simulink model "part2"  (R2025a)
settings: Solver=ode4  StartTime=0.0  StopTime=500  FixedStep=0.1  RelTol=1e-3
values from neighbouring files (symbols this model uses):
  A_f = diag([1/t1 1/t2 1/t3])    [reference_model.m]
  A_w = [zeros(3,3), eye(3); -omega_ekf^2, -2*lambda_ekf*omega_ekf]    [kalman.m]
  Aw = [zeros(3,3), eye(3); -omega*omega, -2*lambda*omega]    [observer.m]
  B_ekf = [zeros(6,3);zeros(3,3); zeros(3,3);M_inv]    [kalman.m]
  Cw = [zeros(3,3), eye(3)]    [observer.m]
  D_diag = D    [observer.m]
  E_ekf = [E_w zeros(6,3) ... (first row only)    [kalman.m]
  G = zeros(3,3)    [kalman.m]
  Gamma = diag([w1^2, w2^2, w3^2])    [reference_model.m]
  H_ekf = [C_w eye(3) zeros(3,3) zeros(3,3)]    [kalman.m]
  h_ekf = 0.1    [kalman.m]
  K1 = [diag([k1, k2, k3]); diag([k4, k5, k6])]    [observer.m]
  K2 = diag([k7, k8, k9])    [observer.m]
  K3 = 0.1* K4    [observer.m]
  K4 = diag([M_diag(1,1), M_diag(1,1), M_diag(1,1)])*1e-1    [observer.m]
  K_w_ekf = diag(Kwi)    [kalman.m]
  Kd = diag([Kd_t(1,1), Kd_t(2,2), Kd_t(3,3)])    [PID.m]
  Ki = diag([Ki_t(1,1), Ki_t(2,2), Ki_t(3,3)])    [PID.m]
  Kp = diag([Kp_t(1,1), Kp_t(2,2), Kp_t(3,3)])    [PID.m]
  lambda_ekf = diag(zeta)    [kalman.m]
  M_diag = [Mtot(1,1), 0, 0 ... (first row only)    [observer.m]
  M_inv = inv(M_3)    [kalman.m]    (also in observer.m = inv(M_diag))
  mu = 0.001    [init.m]
  mu_direction = 0.03    [init.m]
  Omega = diag([2*zeta1*w1, 2*zeta2*w2, 2*zeta3*w3])    [reference_model.m]
  omega_ekf = diag([w, w, w])    [kalman.m]
  P_0 = eye(15)    [kalman.m]
  Q_ekf = diag([0.001, 0.001, 0.001, 1e8, 1e8, 1e9])    [kalman.m]
  R_ekf = diag([1, 5, 0.01])    [kalman.m]
  rate = [rate(1), rate(2), rate(2), rate(3), rate(4),rate(4), rate(5), rate(5)]    [thrust_allocation.m]
  rotationspeed = [0 rotationspeed(1) 0 rotationspeed(2) rotationspeed(3)]    [thrust_allocation.m]
  step1 = 50    [reference_model.m]
  step2 = 1.4    [reference_model.m]
  step3 = 1.2    [reference_model.m]
  T_b_ekf = 1000*diag([1, 1, 1])    [kalman.m]
  Tb_inv = inv(Tb)    [observer.m]
  thrust = [thrust(1), thrust(2), thrust(2), thrust(3), thrust(4), thrust(4), thrust(5), thrust(5)]    [thrust_allocation.m]
  U_10 = 10    [init.m]
  U_angle = 180    [init.m]
  U_mean = U_10*(5/2)*sqrt(K)*log(z/z0)    [init.m]
  W = diag([10, 1, 1, 10, 1, 1, 1, 1])    [thrust_allocation.m]
  w = 0.005    [init.m]    (also in kalman.m = 0.698131700798)
  x_0 = zeros(1,15)    [kalman.m]
  xpos = [thrusters.xposition]    [thrust_allocation.m]
  ypos = [thrusters.yposition]    [thrust_allocation.m]
undefined symbols (not defined in the file or in its folder): alpha, C_pitch, C_roll, C_yaw, Cx, Cy, Cz, Hoerner, thrusters, vessel, wind_coeff
libraries: marine_gnc x9, simulink x8, dspsigops x3, marine_hydro x2, simulink_extras x2
(part 1 of 2)
settings Model: Creator=jonbjor  LastModifiedBy=audun
settings DataIOCC: ReturnWorkspaceOutputs=off
settings DebuggingCC: AlgebraicLoopMsg=none  UnconnectedInputMsg=warning  UnconnectedOutputMsg=warning  UnconnectedLineMsg=warning  ArithmeticOperatorsInVariantConditions=warning
settings ModelReferenceCC: EnableRefExpFcnMdlSchedulingChecks=on
settings SFSimCC: SimUseLocalCustomCode=off  CustomCodeUndefinedFunction=UseInterfaceOnly
settings RTWCC: RTWUseLocalCustomCode=off  GPUComputeCapability=3.5  DLArmComputeVersion=19.05

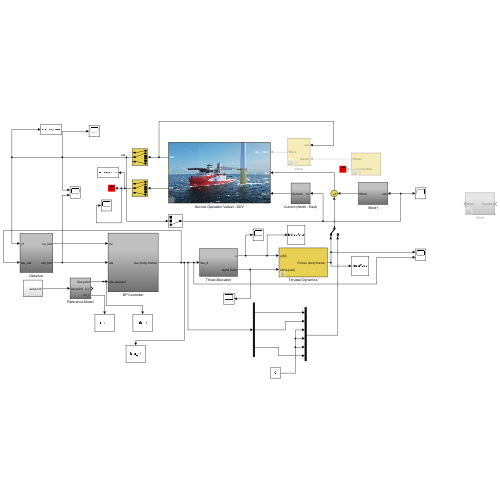
[thumbnail: Simulink's stored preview of the top-level diagram]
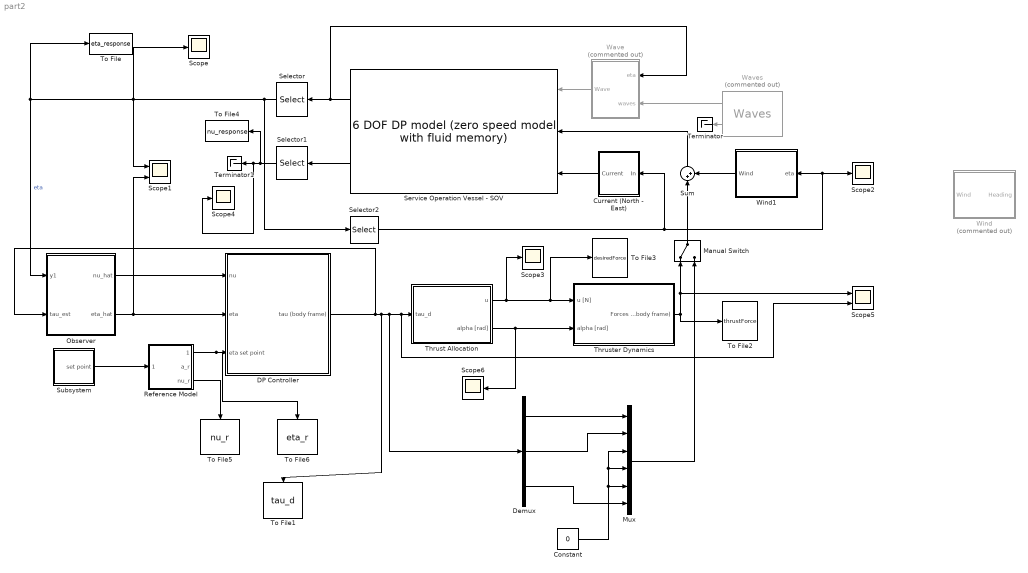
== system part2 ==
  Constant : Constant  Value=0
  Current (North - East) : Subsystem
  DP Controller : Subsystem
  Demux : Demux  Outputs=3
  Manual Switch : ManualSwitch
  Mux : Mux  Inputs=6
  Observer : Subsystem
  Reference Model : Subsystem
  Scope{,2..4,6} (5 alike) : Scope
      Scope settings: ActiveDisplayYMinimum=-447.3734  ActiveDisplayYMaximum=52.18517  DataLoggingVariableName=ScopeData6
      Scope2 settings: ActiveDisplayYMinimum=-0.38407  ActiveDisplayYMaximum=3.45663  DataLoggingVariableName=ScopeData2
      Scope3 settings: ActiveDisplayYMinimum=-11170.42553  ActiveDisplayYMaximum=24574.49173
      Scope4 settings: ActiveDisplayYMinimum=-1.13887  ActiveDisplayYMaximum=0.80341  DataLoggingVariableName=ScopeData2
      Scope6 settings: ActiveDisplayYMinimum=-0.17279  ActiveDisplayYMaximum=1.76453
  Scope1 : Scope  NumInputPorts=2
      settings: ActiveDisplayYMinimum=-560.03158  ActiveDisplayYMaximum=66.18767
  Scope5 : Scope  NumInputPorts=2
      settings: ActiveDisplayYMinimum=-36332.60871  ActiveDisplayYMaximum=326993.47836  DataLoggingVariableName=ScopeData3
  Selector : Selector  InputPortWidth=6  IndexOptions=Index vector (dialog)  Indices=[1 2 6]  OutputSizes=1
  Selector1 : Selector  InputPortWidth=6  IndexOptions=Index vector (dialog)  Indices=[1 2 6]  OutputSizes=1
  Selector2 : Selector  InputPortWidth=3  IndexOptions=Index vector (dialog)  Indices=[3]  OutputSizes=1
  Service Operation Vessel - SOV : marine_hydro/Hydro Library/6 DOF DP model  (zero speed model with fluid memory)  ABC=vesselABC  rho=1025  Axc=0.9*vessel.main.T*vessel.main.B  Ayc=0.9*vessel.main.T*vessel.main.Lpp  CX=1  CY_2D=Hoerner(vessel.main.B,vessel.main.T)  Bv=vessel.Bv  mask(6 DOF zero speed model){}
      link override "Integrator1 ": InitialCondition=nu0
      link override Integrator2: InitialCondition=eta0
      settings: SourceProductName=MSS Hydro
      mask Display:
      | image('SOV.jpg');
      | color('white'); port_label('output', 1, 'eta')
      | color('white'); port_label('output', 2, 'nu')
      | color('white'); port_label('input', 1, 'tau_wave')
      | color('white'); port_label('input', 2, 'tau')
      | color('white'); port_label('input', 3, 'nu_c')
  Subsystem : Subsystem
  Sum : Sum  Inputs=|++
  Terminator : Terminator
  Terminator1 : Terminator
  Thrust Allocation : Subsystem
  Thruster Dynamics : Subsystem  mask{thrusterfault=off}
      mask prompts: thrusterfault "Fault on thruster #2 and #4?"
  To File : ToFile  Filename=eta_response  MatrixName=eta_response
  To File1 : ToFile  Filename=tau_d  MatrixName=tau_d
  To File2 : ToFile  Filename=thrustForce  MatrixName=thrustForce
  To File3 : ToFile  Filename=desiredForce  MatrixName=desiredForce
  To File4 : ToFile  Filename=nu_response  MatrixName=nu_response
  To File5 : ToFile  Filename=nu_r  MatrixName=nu_r
  To File6 : ToFile  Filename=eta_r  MatrixName=eta_r
  Wave : Subsystem  Commented=on  mask{waveforces=on}
      mask prompts: waveforces "Waveforces enabled"
  Waves : marine_gnc/Environment/Waves/Waves  Commented=on  spectrum_type=ITTC  disp_flag=on  plot_spectrum=off  plot_realization=off  hs=2.5  omega_peak=2*pi/9  psi_mean=0  gamma=-1  spread=2  depth=inf  nfreq=20  ndir=10  energylim=0.005  freq_cutoff=3  dir_cutoff=0  rand_seed=123  rand_freq=on  rand_dir=on  Zeta_a=0  Omega=0  Phase=0  Wavenum=0  Psi=0
      link override Psi: Value=-6*pi/8*ones(1,38)
      settings: SourceProductName=MSS GNC
  Wind : Subsystem  Commented=on
  Wind1 : Subsystem
  wires:
  Service Operation Vessel - SOV/2 -> Selector1/1
  Service Operation Vessel - SOV/1 -> Wave/1(eta), Selector/1
  Current (North - East)/1(Current) -> Service Operation Vessel - SOV/3
  Wave/1(Wave) -> Service Operation Vessel - SOV/1
  Waves/1 -> Wave/2(waves)
  Waves/2 -> Terminator/1
  Sum/1 -> Service Operation Vessel - SOV/2
  Selector/1 -> Selector2/1, Scope/1, To File/1, Observer/1(y1), Scope1/1  "eta"
  Reference Model/1(Set-point) -> To File6/1, DP Controller/3(eta set point)
  Subsystem/1(set point) -> Reference Model/1(set point)
  Selector2/1 -> Wind1/1(eta), Scope2/1, Current (North - East)/1(In)
  Observer/2(eta_hat) -> DP Controller/2(eta), Scope1/2
  Demux/1 -> Mux/1
  Demux/2 -> Mux/2
  Demux/3 -> Mux/6
  Constant/1 -> Mux/4, Mux/3, Mux/5
  Selector1/1 -> To File4/1, Scope4/1, Terminator1/1
  Mux/1 -> Manual Switch/2
  Thruster Dynamics/1("Forces (body frame) ") -> Manual Switch/1, Scope5/1, To File2/1
  Thrust Allocation/2(alpha [rad]) -> Scope6/1, Thruster Dynamics/2(alpha [rad])
  Thrust Allocation/1(u) -> To File3/1, Thruster Dynamics/1(u [N]), Scope3/1
  Wind1/1(Wind) -> Sum/2
  Reference Model/3(nu_r) -> To File5/1
  Manual Switch/1 -> Sum/1
  Observer/1(nu_hat) -> DP Controller/1(nu)
  DP Controller/1(tau (body frame)) -> Scope5/2, Thrust Allocation/1(tau_d), Demux/1, To File1/1, Observer/2(tau_est)

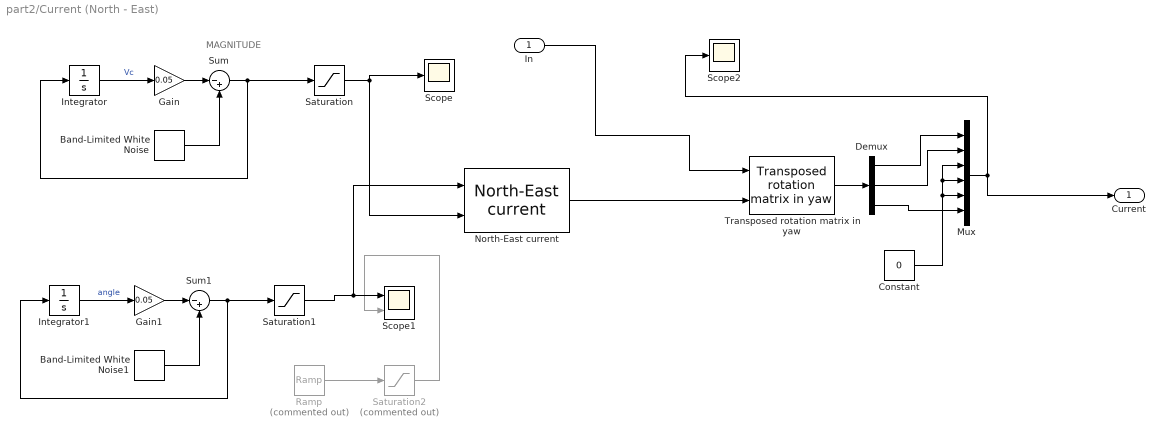
== system part2/Current (North - East) ==
  note: MAGNITUDE
  In : Inport
  Band-Limited White Noise : simulink/Sources/Band-Limited White Noise  Cov=[0.1]  Ts=0.1  seed=[23341]
  Band-Limited White Noise1 : simulink/Sources/Band-Limited White Noise  Cov=[0.1]  Ts=0.1  seed=[23341]
  Constant : Constant  Value=0
  Demux : Demux  Outputs=3
  Gain : Gain  Gain=0.05
  Gain1 : Gain  Gain=0.05
  Integrator : Integrator
  Integrator1 : Integrator
  Mux : Mux  Inputs=6
  North-East current : marine_gnc/Environment/Current/North-East current  SystemSampleTime=-1  VariantActivationTime=update diagram  EmptyChoice=off  PassThrough=off  PassThroughVariantControl=(default)  EmptyChoiceVariantControl=(default)  AllowFlexibleInterface=on  Latency=0  AutoFrameSizeCalculation=off
      settings: SourceProductName=MSS GNC
  Ramp : simulink/Sources/Ramp  Commented=on  slope=0.3  start=0  InitialOutput=180
  Saturation : Saturate  UpperLimit=0.2  LowerLimit=0.2
  Saturation1 : Saturate  UpperLimit=270  LowerLimit=270
  Saturation2 : Saturate  Commented=on  UpperLimit=270  LowerLimit=0
  Scope : Scope
      settings: ActiveDisplayYMinimum=0.4  ActiveDisplayYMaximum=0.6  DataLoggingVariableName=ScopeData2
  Scope1 : Scope  NumInputPorts=2
      settings: ActiveDisplayYMinimum=-33.75  ActiveDisplayYMaximum=303.75  DataLoggingVariableName=ScopeData3
  Scope2 : Scope
      settings: ActiveDisplayYMinimum=-0.22527  ActiveDisplayYMaximum=0.02745  DataLoggingVariableName=ScopeData4
  Sum : Sum  Inputs=|-+
  Sum1 : Sum  Inputs=|-+
  Transposed rotation matrix in yaw : marine_gnc/Models/ Kinematics/Transposed rotation  matrix in yaw
      settings: SourceProductName=MSS GNC
  Current : Outport  VectorParamsAs1DForOutWhenUnconnected=off
  wires:
  Demux/3 -> Mux/6
  Band-Limited White Noise/1 -> Sum/2
  North-East current/1 -> Transposed rotation matrix in yaw/2
  Integrator1/1 -> Gain1/1  "angle"
  Saturation/1 -> Scope/1, North-East current/2
  Ramp/1 -> Saturation2/1
  Mux/1 -> Current/1, Scope2/1
  Saturation2/1 -> Scope1/2
  Saturation1/1 -> North-East current/1, Scope1/1
  Gain1/1 -> Sum1/1
  Integrator/1 -> Gain/1  "Vc"
  In/1 -> Transposed rotation matrix in yaw/1
  Sum1/1 -> Saturation1/1, Integrator1/1
  Gain/1 -> Sum/1
  Constant/1 -> Mux/5, Mux/4, Mux/3
  Demux/2 -> Mux/2
  Transposed rotation matrix in yaw/1 -> Demux/1
  Sum/1 -> Saturation/1, Integrator/1
  Band-Limited White Noise1/1 -> Sum1/2
  Demux/1 -> Mux/1

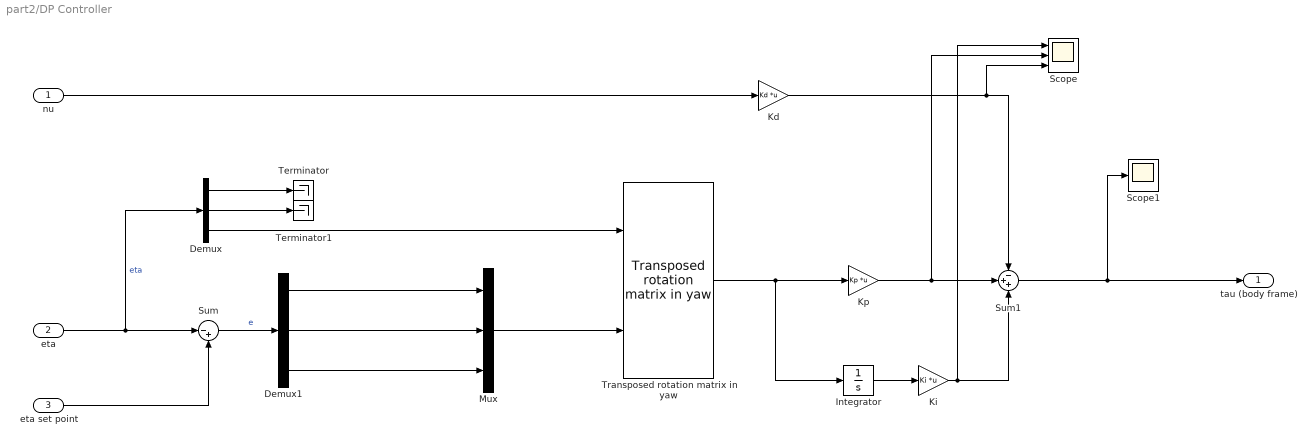
== system part2/DP Controller ==
  nu : Inport
  eta : Inport  Port=2
  eta set point : Inport  Port=3
  Demux : Demux  Outputs=3
  Demux1 : Demux  Outputs=3
  Integrator : Integrator
  Kd : Gain  Gain=Kd  Multiplication=Matrix(K*u)
  Ki : Gain  Gain=Ki  Multiplication=Matrix(K*u)
  Kp : Gain  Gain=Kp  Multiplication=Matrix(K*u)
  Mux : Mux  Inputs=3
  Scope : Scope  NumInputPorts=3
      settings: ActiveDisplayYMinimum=-4.19221098515E+6  ActiveDisplayYMaximum=1.94440858121E+6
  Scope1 : Scope
      settings: ActiveDisplayYMinimum=-1.437861965646E+7  ActiveDisplayYMaximum=4.290926657906E+7
  Sum : Sum  Inputs=|-+
  Sum1 : Sum  Inputs=-++
  Terminator : Terminator
  Terminator1 : Terminator
  Transposed rotation matrix in yaw : marine_gnc/Models/ Kinematics/Transposed rotation  matrix in yaw
      settings: SourceProductName=MSS GNC
  tau (body frame) : Outport  VectorParamsAs1DForOutWhenUnconnected=off
  wires:
  Demux/2 -> Terminator1/1
  nu/1 -> Kd/1
  Transposed rotation matrix in yaw/1 -> Integrator/1, Kp/1
  Kp/1 -> Scope/2, Sum1/2
  Sum1/1 -> Scope1/1, tau (body frame)/1
  Mux/1 -> Transposed rotation matrix in yaw/2
  Demux1/2 -> Mux/2
  Demux1/1 -> Mux/1
  Kd/1 -> Scope/3, Sum1/1
  Demux/1 -> Terminator/1
  Ki/1 -> Scope/1, Sum1/3
  Sum/1 -> Demux1/1  "e"
  eta/1 -> Demux/1, Sum/1  "eta"
  Integrator/1 -> Ki/1
  eta set point/1 -> Sum/2
  Demux/3 -> Transposed rotation matrix in yaw/1
  Demux1/3 -> Mux/3

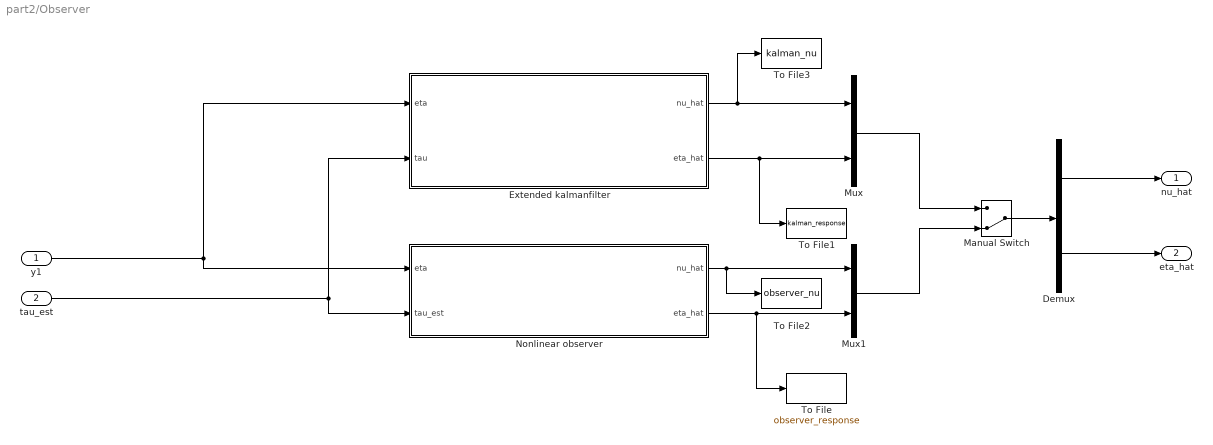
== system part2/Observer ==
  y1 : Inport
  tau_est : Inport  Port=2
  Demux : Demux  Outputs=2
  Extended kalmanfilter : Subsystem
  Manual Switch : ManualSwitch  CurrentSetting=0
  Mux : Mux  Inputs=2
  Mux1 : Mux  Inputs=2
  Nonlinear observer : Subsystem
  To File : ToFile  Filename=observer_response  MatrixName=eta_observer
  To File1 : ToFile  Filename=kalman_response  MatrixName=eta_kalman
  To File2 : ToFile  Filename=observer_nu  MatrixName=nu_observer
  To File3 : ToFile  Filename=kalman_nu  MatrixName=nu_kalman
  nu_hat : Outport  VectorParamsAs1DForOutWhenUnconnected=off
  eta_hat : Outport  Port=2  VectorParamsAs1DForOutWhenUnconnected=off
  wires:
  y1/1 -> Extended kalmanfilter/1(eta), Nonlinear observer/1(eta)
  tau_est/1 -> Extended kalmanfilter/2(tau), Nonlinear observer/2(tau_est)
  Extended kalmanfilter/2(eta_hat) -> To File1/1, Mux/2
  Extended kalmanfilter/1(nu_hat) -> To File3/1, Mux/1
  Nonlinear observer/2(eta_hat) -> To File/1, Mux1/2
  Nonlinear observer/1(nu_hat) -> To File2/1, Mux1/1
  Mux1/1 -> Manual Switch/2
  Mux/1 -> Manual Switch/1
  Manual Switch/1 -> Demux/1
  Demux/2 -> eta_hat/1
  Demux/1 -> nu_hat/1

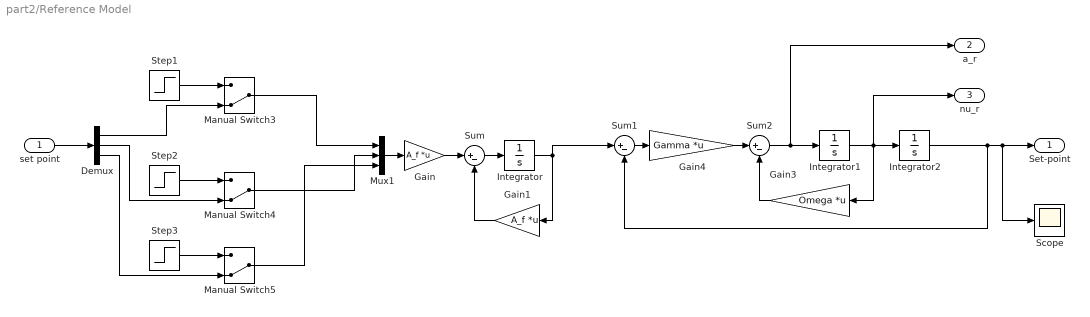
== system part2/Reference Model ==
  set point : Inport
  Demux : Demux  Outputs=3
  Gain : Gain  Gain=A_f  Multiplication=Matrix(K*u)
  Gain1 : Gain  Gain=A_f  Multiplication=Matrix(K*u)
  Gain3 : Gain  Gain=Omega  Multiplication=Matrix(K*u)
  Gain4 : Gain  Gain=Gamma  Multiplication=Matrix(K*u)
  Integrator : Integrator
  Integrator1 : Integrator
  Integrator2 : Integrator
  Manual Switch3 : ManualSwitch  CurrentSetting=0
  Manual Switch4 : ManualSwitch  CurrentSetting=0
  Manual Switch5 : ManualSwitch  CurrentSetting=0
  Mux1 : Mux  Inputs=3
  Scope : Scope
      settings: ActiveDisplayYMinimum=-62.49997  ActiveDisplayYMaximum=62.49997  DataLoggingVariableName=ScopeData5
  Step1 : Step  After=step1  SampleTime=1
  Step2 : Step  After=step2  SampleTime=1
  Step3 : Step  After=step3  SampleTime=1
  Sum : Sum  Inputs=|+-
  Sum1 : Sum  Inputs=|+-
  Sum2 : Sum  Inputs=|+-
  Set-point : Outport  VectorParamsAs1DForOutWhenUnconnected=off
  a_r : Outport  Port=2
  nu_r : Outport  Port=3
  wires:
  set point/1 -> Demux/1
  Mux1/1 -> Gain/1
  Integrator1/1 -> Gain3/1, nu_r/1, Integrator2/1
  Manual Switch5/1 -> Mux1/3
  Gain3/1 -> Sum2/2
  Manual Switch4/1 -> Mux1/2
  Sum2/1 -> a_r/1, Integrator1/1
  Step1/1 -> Manual Switch3/1
  Gain4/1 -> Sum2/1
  Sum1/1 -> Gain4/1
  Step3/1 -> Manual Switch5/1
  Demux/2 -> Manual Switch4/2
  Gain1/1 -> Sum/2
  Sum/1 -> Integrator/1
  Manual Switch3/1 -> Mux1/1
  Demux/1 -> Manual Switch3/2
  Demux/3 -> Manual Switch5/2
  Integrator2/1 -> Sum1/2, Scope/1, Set-point/1
  Gain/1 -> Sum/1
  Step2/1 -> Manual Switch4/1
  Integrator/1 -> Sum1/1, Gain1/1

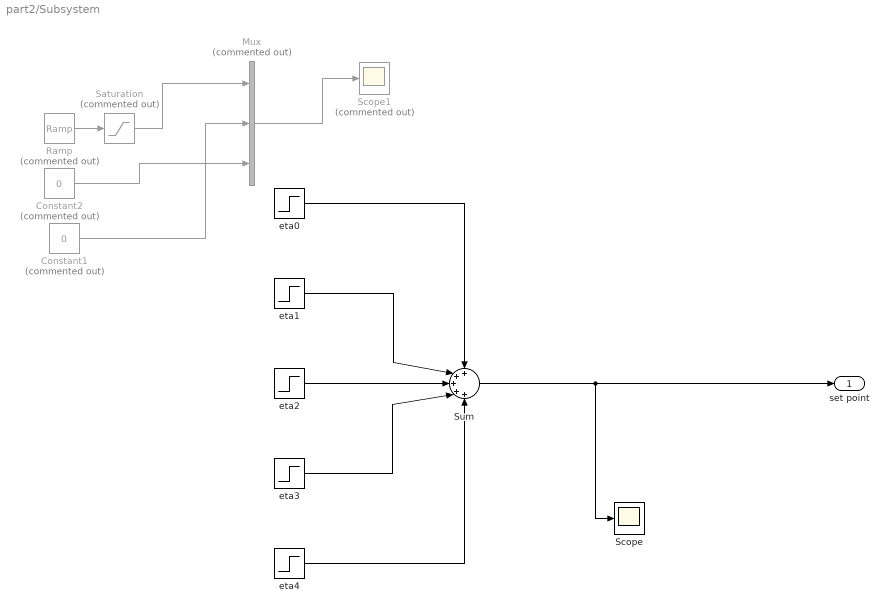
== system part2/Subsystem ==
  Constant1 : Constant  Commented=on  Value=0
  Constant2 : Constant  Commented=on  Value=0
  Mux : Mux  Commented=on  Inputs=3
  Ramp : simulink/Sources/Ramp  Commented=on  slope=0.2  start=0  InitialOutput=0
  Saturation : Saturate  Commented=on  UpperLimit=50  LowerLimit=0
  Scope : Scope
      settings: ActiveDisplayYMinimum=-6.25  ActiveDisplayYMaximum=56.25  DataLoggingVariableName=ScopeData2
  Scope1 : Scope  Commented=on
      settings: ActiveDisplayYMinimum=-6.25  ActiveDisplayYMaximum=56.25
  Sum : Sum  Inputs=+++++
  eta0 : Step  Before=[0, 0 , 0]  After=[50, 0, 0]  SampleTime=0
  eta1 : Step  Time=601  Before=[0, 0 , 0]  After=[0, -50, 0]  SampleTime=0
  eta2 : Step  Time=1201  Before=[0, 0, 0]  After=[0, 0, -pi/4]  SampleTime=0
  eta3 : Step  Time=1801  Before=[0, 0, 0]  After=[-50, 0, 0]  SampleTime=0
  eta4 : Step  Time=2401  Before=[0, 0, 0]  After=[0, 50, pi/4]  SampleTime=0
  set point : Outport
  wires:
  Sum/1 -> set point/1, Scope/1
  eta0/1 -> Sum/1
  eta1/1 -> Sum/2
  eta2/1 -> Sum/3
  eta3/1 -> Sum/4
  eta4/1 -> Sum/5
  Ramp/1 -> Saturation/1
  Constant1/1 -> Mux/2
  Constant2/1 -> Mux/3
  Saturation/1 -> Mux/1
  Mux/1 -> Scope1/1

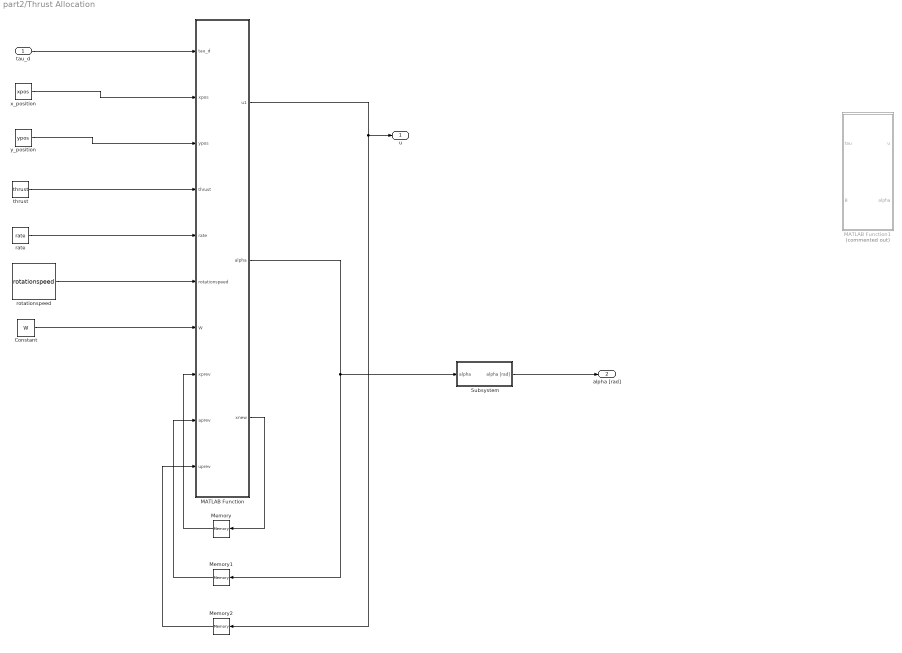
== system part2/Thrust Allocation ==
  tau_d : Inport
  Constant : Constant  Value=W
  MATLAB Function : MATLAB Function  TreatAsAtomicUnit=on
  MATLAB Function1 : MATLAB Function  Commented=on  TreatAsAtomicUnit=on
  Memory : Memory  InitialCondition=zeros(8,1)
  Memory1 : Memory  InitialCondition=zeros(5,1)
  Memory2 : Memory  InitialCondition=zeros(5,1)
  Subsystem : Subsystem
  rate : Constant  Value=rate
  rotationspeed : Constant  Value=rotationspeed
  thrust : Constant  Value=thrust
  x_position : Constant  Value=xpos
  y_position : Constant  Value=ypos
  u : Outport  VectorParamsAs1DForOutWhenUnconnected=off
  alpha [rad] : Outport  Port=2  VectorParamsAs1DForOutWhenUnconnected=off
  wires:
  y_position/1 -> MATLAB Function/3(ypos)
  MATLAB Function/1(u1) -> Memory2/1, u/1
  MATLAB Function/2(alpha) -> Memory1/1, Subsystem/1(alpha)
  rate/1 -> MATLAB Function/5(rate)
  tau_d/1 -> MATLAB Function/1(tau_d)
  x_position/1 -> MATLAB Function/2(xpos)
  Constant/1 -> MATLAB Function/7(W)
  rotationspeed/1 -> MATLAB Function/6(rotationspeed)
  thrust/1 -> MATLAB Function/4(thrust)
  MATLAB Function/3(xnew) -> Memory/1
  Memory/1 -> MATLAB Function/8(xprev)
  Memory1/1 -> MATLAB Function/9(aprev)
  Memory2/1 -> MATLAB Function/10(uprev)
  Subsystem/1(alpha [rad]) -> alpha [rad]/1

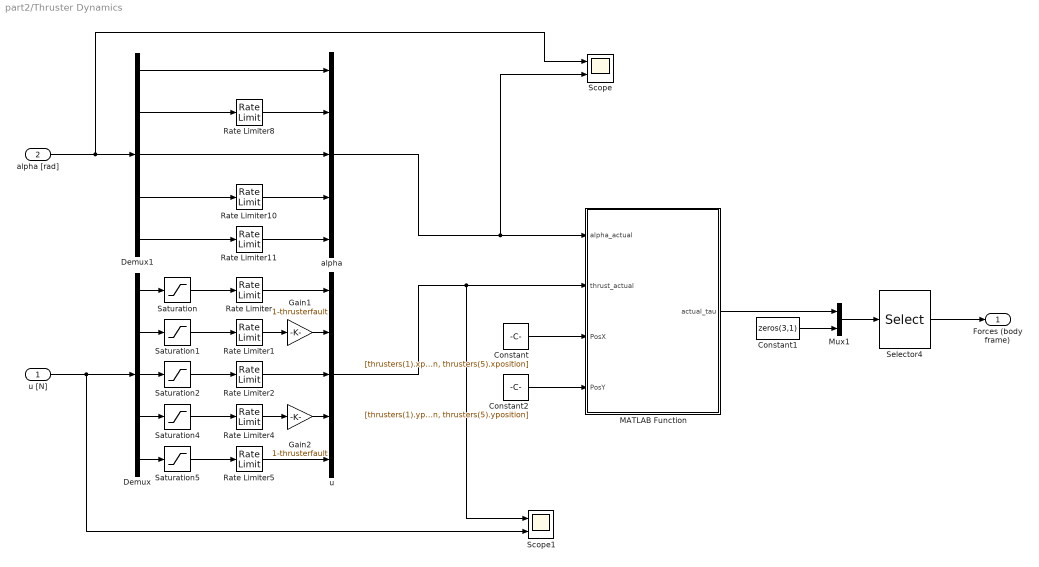
== system part2/Thruster Dynamics ==
  u [N] : Inport
  alpha [rad] : Inport  Port=2
  Constant : Constant  Value=[thrusters(1).xposition, thrusters(2).xposition, thrusters(3).xposition, thrusters(4).xposition, thrusters(5).xposition]
  Constant1 : Constant  Value=zeros(3,1)
  Constant2 : Constant  Value=[thrusters(1).yposition, thrusters(2).yposition, thrusters(3).yposition, thrusters(4).yposition, thrusters(5).yposition]
  Demux : Demux  Outputs=5
  Demux1 : Demux  Outputs=5
  Gain1 : Gain  Gain=1-thrusterfault
  Gain2 : Gain  Gain=1-thrusterfault
  MATLAB Function : MATLAB Function  TreatAsAtomicUnit=on
  Mux1 : Mux  Inputs=2
  Rate Limiter : RateLimiter  RisingSlewLimit=thrusters(1).rate  FallingSlewLimit=-thrusters(1).rate  SampleTimeMode=inherited
  Rate Limiter1 : RateLimiter  RisingSlewLimit=thrusters(2).rate  FallingSlewLimit=-thrusters(2).rate  SampleTimeMode=inherited
  Rate Limiter10 : RateLimiter  RisingSlewLimit=thrusters(4).rotationspeed  FallingSlewLimit=-thrusters(4).rotationspeed  SampleTimeMode=inherited
  Rate Limiter11 : RateLimiter  RisingSlewLimit=thrusters(5).rotationspeed  FallingSlewLimit=-thrusters(5).rotationspeed  SampleTimeMode=inherited
  Rate Limiter2 : RateLimiter  RisingSlewLimit=thrusters(3).rate  FallingSlewLimit=-thrusters(3).rate  SampleTimeMode=inherited
  Rate Limiter4 : RateLimiter  RisingSlewLimit=thrusters(4).rate  FallingSlewLimit=-thrusters(4).rate  SampleTimeMode=inherited
  Rate Limiter5 : RateLimiter  RisingSlewLimit=thrusters(5).rate  FallingSlewLimit=-thrusters(5).rate  SampleTimeMode=inherited
  Rate Limiter8 : RateLimiter  RisingSlewLimit=thrusters(2).rotationspeed  FallingSlewLimit=-thrusters(2).rotationspeed  SampleTimeMode=inherited
  Saturation : Saturate  UpperLimit=thrusters(1).thrust  LowerLimit=-thrusters(1).thrust
  Saturation1 : Saturate  UpperLimit=thrusters(2).thrust  LowerLimit=-thrusters(2).thrust
  Saturation2 : Saturate  UpperLimit=thrusters(3).thrust  LowerLimit=-thrusters(3).thrust
  Saturation4 : Saturate  UpperLimit=thrusters(4).thrust  LowerLimit=-thrusters(4).thrust
  Saturation5 : Saturate  UpperLimit=thrusters(5).thrust  LowerLimit=-thrusters(5).thrust
  Scope : Scope  NumInputPorts=2
      settings: ActiveDisplayYMinimum=-4.84885  ActiveDisplayYMaximum=3.59264  DataLoggingVariableName=ScopeData4
  Scope1 : Scope  NumInputPorts=2
      settings: ActiveDisplayYMinimum=-375000  ActiveDisplayYMaximum=375000  DataLoggingVariableName=ScopeData5
  Selector4 : Selector  InputPortWidth=6  IndexOptions=Index vector (dialog)  Indices=[1 2 4 5 6 3]  OutputSizes=1
  alpha : Mux  Inputs=5
  u : Mux  Inputs=5
  "Forces (body frame) " : Outport  VectorParamsAs1DForOutWhenUnconnected=off
  wires:
  Rate Limiter2/1 -> u/3
  Saturation/1 -> Rate Limiter/1
  Mux1/1 -> Selector4/1
  Constant1/1 -> Mux1/2
  Saturation4/1 -> Rate Limiter4/1
  Demux/2 -> Saturation1/1
  Saturation1/1 -> Rate Limiter1/1
  Demux/1 -> Saturation/1
  Demux/3 -> Saturation2/1
  Saturation2/1 -> Rate Limiter2/1
  Selector4/1 -> "Forces (body frame) "/1
  Gain1/1 -> u/2
  Rate Limiter1/1 -> Gain1/1
  Rate Limiter/1 -> u/1
  Rate Limiter4/1 -> Gain2/1
  Saturation5/1 -> Rate Limiter5/1
  u [N]/1 -> Scope1/2, Demux/1
  alpha [rad]/1 -> Scope/1, Demux1/1
  Constant/1 -> MATLAB Function/3(PosX)
  Constant2/1 -> MATLAB Function/4(PosY)
  u/1 -> Scope1/1, MATLAB Function/2(thrust_actual)
  alpha/1 -> Scope/2, MATLAB Function/1(alpha_actual)
  MATLAB Function/1(actual_tau) -> Mux1/1
  Rate Limiter10/1 -> alpha/4
  Demux1/4 -> Rate Limiter10/1
  Demux1/5 -> Rate Limiter11/1
  Rate Limiter11/1 -> alpha/5
  Demux1/1 -> alpha/1
  Gain2/1 -> u/4
  Demux/4 -> Saturation4/1
  Demux/5 -> Saturation5/1
  Rate Limiter5/1 -> u/5
  Demux1/2 -> Rate Limiter8/1
  Rate Limiter8/1 -> alpha/2
  Demux1/3 -> alpha/3

== system part2/Wave ==
  eta : Inport
  waves : Inport  Port=2
  Gain : Gain  Gain=waveforces
  Sum : Sum
  Wave loads (U=0) : marine_hydro/Hydro Library/Wave loads (U=0)  SystemSampleTime=-1  VariantActivationTime=update diagram  AllowFlexibleInterface=on  Latency=0  AutoFrameSizeCalculation=off
      settings: SourceProductName=MSS Hydro
  Wave : Outport  VectorParamsAs1DForOutWhenUnconnected=off
  wires:
  eta/1 -> Wave loads (U=0)/1
  waves/1 -> Wave loads (U=0)/2
  Sum/1 -> Gain/1
  Wave loads (U=0)/1 -> Sum/1
  Wave loads (U=0)/2 -> Sum/2
  Gain/1 -> Wave/1

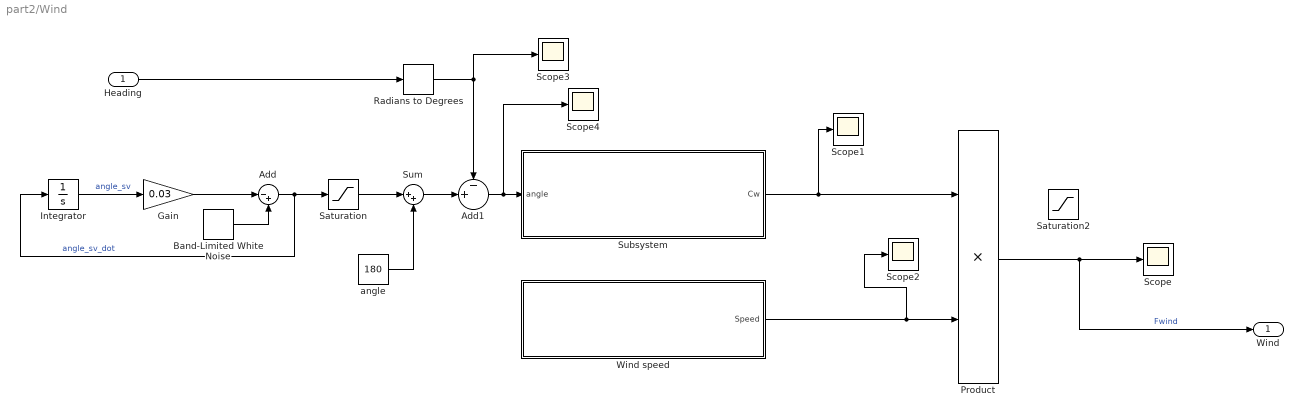
== system part2/Wind ==
  Heading : Inport
  Add : Sum  Inputs=|-+
  Add1 : Sum  Inputs=-+|
  Band-Limited White Noise : simulink/Sources/Band-Limited White Noise  Cov=[0.005]  Ts=0.1  seed=[23381]
  Gain : Gain  Gain=0.03
  Integrator : Integrator
  Product : Product
  Radians to Degrees : simulink_extras/Transformations/Radians to Degrees
  Saturation : Saturate  UpperLimit=5  LowerLimit=-5
  Saturation2 : Saturate  UpperLimit=1.5e7  LowerLimit=-1.5e7
  Scope{,1..4} (5 alike) : Scope
      Scope settings: ActiveDisplayYMinimum=-1.182594251627E+7  ActiveDisplayYMaximum=8.065927737314E+7
      Scope1 settings: ActiveDisplayYMinimum=-91004.06859  ActiveDisplayYMaximum=620694.24596
      Scope2 settings: ActiveDisplayYMinimum=-1.88941  ActiveDisplayYMaximum=161.7268  DataLoggingVariableName=ScopeData3
      Scope3 settings: ActiveDisplayYMinimum=-22.00561  ActiveDisplayYMaximum=198.05046  DataLoggingVariableName=ScopeData2
      Scope4 settings: ActiveDisplayYMinimum=-18.34813  ActiveDisplayYMaximum=202.39104  DataLoggingVariableName=ScopeData4
  Subsystem : Subsystem
  Sum : Sum  Inputs=|++
  Wind speed : Subsystem
  angle : Constant  Value=180
  Wind : Outport  VectorParamsAs1DForOutWhenUnconnected=off
  wires:
  Wind speed/1(Speed) -> Scope2/1, Product/2
  Product/1 -> Wind/1, Scope/1  "Fwind"
  Integrator/1 -> Gain/1  "angle_sv"
  Gain/1 -> Add/1
  Band-Limited White Noise/1 -> Add/2
  Add/1 -> Integrator/1, Saturation/1  "angle_sv_dot"
  Subsystem/1(Cw) -> Scope1/1, Product/1
  Saturation/1 -> Sum/1
  angle/1 -> Sum/2
  Sum/1 -> Add1/2
  Add1/1 -> Scope4/1, Subsystem/1(angle)
  Radians to Degrees/1 -> Scope3/1, Add1/1
  Heading/1 -> Radians to Degrees/1

== system part2/Wind1 ==
  eta : Inport
  Product : Product
  Scope : Scope
      settings: ActiveDisplayYMinimum=-10.58446  ActiveDisplayYMaximum=229.08832  DataLoggingVariableName=ScopeData2
  Scope1 : Scope
      settings: ActiveDisplayYMinimum=-7902.64806  ActiveDisplayYMaximum=3071.9609  DataLoggingVariableName=ScopeData3
  Wind direction : Subsystem
  Wind velocity components : Subsystem
  Wind : Outport  VectorParamsAs1DForOutWhenUnconnected=off
  wires:
  eta/1 -> Wind direction/1(eta)
  Wind direction/1(C_w) -> Scope1/1, Product/1
  Wind velocity components/1(U_total) -> Scope/1, Product/2  "U_total"
  Product/1 -> Wind/1

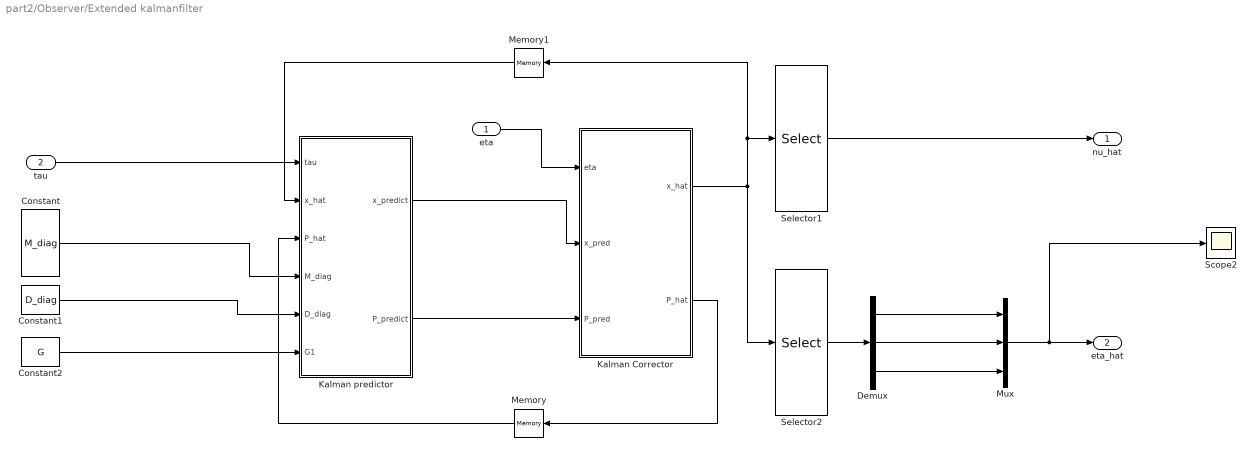
== system part2/Observer/Extended kalmanfilter ==
  eta : Inport
  tau : Inport  Port=2
  Constant : Constant  Value=M_diag
  Constant1 : Constant  Value=D_diag
  Constant2 : Constant  Value=G
  Demux : Demux  Outputs=3
  Kalman Corrector : MATLAB Function  TreatAsAtomicUnit=on
  Kalman predictor : MATLAB Function  TreatAsAtomicUnit=on
  Memory : Memory  InitialCondition=P_0
  Memory1 : Memory  InitialCondition=x_0
  Mux : Mux  Inputs=3
  Scope2 : Scope
      settings: ActiveDisplayYMinimum=-78.08034  ActiveDisplayYMaximum=69.44946
  Selector1 : Selector  InputPortWidth=15  IndexOptions=Index vector (dialog)  Indices=[13 14 15]  OutputSizes=1
  Selector2 : Selector  InputPortWidth=15  IndexOptions=Index vector (dialog)  Indices=[7 8 9]  OutputSizes=1
  nu_hat : Outport
  eta_hat : Outport  Port=2
  wires:
  Memory/1 -> Kalman predictor/3(P_hat)
  Kalman Corrector/1(x_hat) -> Memory1/1, Selector1/1, Selector2/1
  Kalman Corrector/2(P_hat) -> Memory/1
  tau/1 -> Kalman predictor/1(tau)
  Constant1/1 -> Kalman predictor/5(D_diag)
  Constant2/1 -> Kalman predictor/6(G1)
  eta/1 -> Kalman Corrector/1(eta)
  Selector1/1 -> nu_hat/1
  Memory1/1 -> Kalman predictor/2(x_hat)
  Constant/1 -> Kalman predictor/4(M_diag)
  Kalman predictor/1(x_predict) -> Kalman Corrector/2(x_pred)
  Kalman predictor/2(P_predict) -> Kalman Corrector/3(P_pred)
  Demux/1 -> Mux/1
  Selector2/1 -> Demux/1
  Demux/3 -> Mux/3
  Demux/2 -> Mux/2
  Mux/1 -> Scope2/1, eta_hat/1

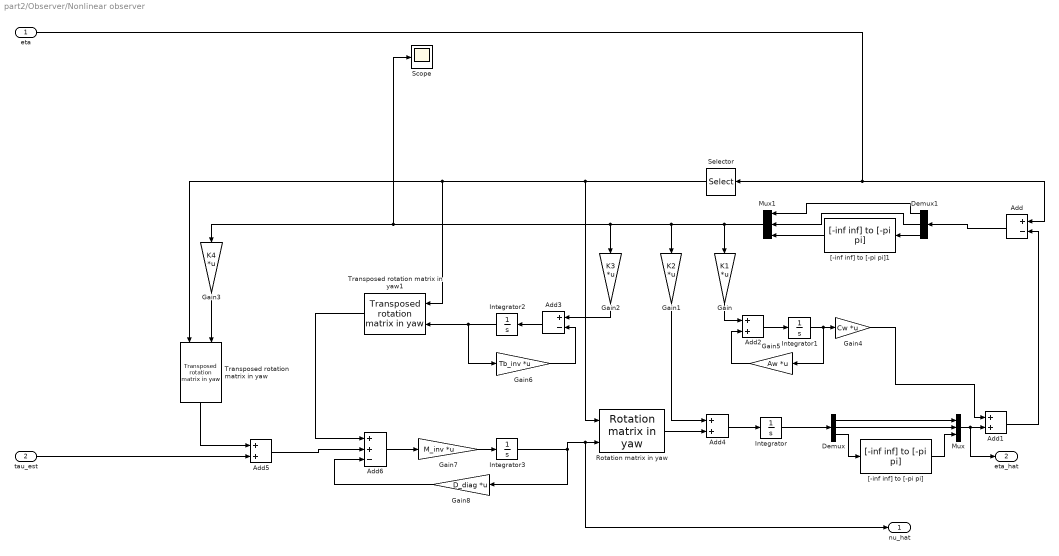
== system part2/Observer/Nonlinear observer ==
  eta : Inport
  tau_est : Inport  Port=2
  Add : Sum  Inputs=+-
  Add{1..2,4..5} (4 alike) : Sum
  Add3 : Sum  Inputs=+-
  Add6 : Sum  Inputs=++-
  Demux : Demux  Outputs=3
      settings: DisplayOption=none
  Demux1 : Demux  Outputs=3
      settings: DisplayOption=none
  Gain : Gain  Gain=K1  Multiplication=Matrix(K*u)
  Gain1 : Gain  Gain=K2  Multiplication=Matrix(K*u)
  Gain2 : Gain  Gain=K3  Multiplication=Matrix(K*u)
  Gain3 : Gain  Gain=K4  Multiplication=Matrix(K*u)
  Gain4 : Gain  Gain=Cw  Multiplication=Matrix(K*u)
  Gain5 : Gain  Gain=Aw  Multiplication=Matrix(K*u)
  Gain6 : Gain  Gain=Tb_inv  Multiplication=Matrix(K*u)
  Gain7 : Gain  Gain=M_inv  Multiplication=Matrix(K*u)
  Gain8 : Gain  Gain=D_diag  Multiplication=Matrix(K*u)
  Integrator{,1..3} (4 alike) : Integrator
  Mux : Mux  Inputs=3
  Mux1 : Mux  Inputs=3
  "Rotation matrix in yaw " : marine_gnc/Models/ Kinematics/Rotation matrix in yaw 
      settings: SourceProductName=MSS GNC
  Scope : Scope
      settings: ActiveDisplayYMinimum=-1.36375  ActiveDisplayYMaximum=3.49816  DataLoggingVariableName=ScopeData2
  Selector : Selector  InputPortWidth=3  IndexOptions=Index vector (dialog)  Indices=[3]  OutputSizes=1
  Transposed rotation matrix in yaw : marine_gnc/Models/ Kinematics/Transposed rotation  matrix in yaw
      settings: SourceProductName=MSS GNC
  Transposed rotation matrix in yaw1 : marine_gnc/Models/ Kinematics/Transposed rotation  matrix in yaw
      settings: SourceProductName=MSS GNC
  "[-inf inf] to [-pi pi]" : marine_gnc/Utilities/Math Operations/[-inf inf] to [-pi pi]
      settings: SourceProductName=MSS GNC
  "[-inf inf] to [-pi pi]1" : marine_gnc/Utilities/Math Operations/[-inf inf] to [-pi pi]
      settings: SourceProductName=MSS GNC
  nu_hat : Outport  VectorParamsAs1DForOutWhenUnconnected=off
  eta_hat : Outport  Port=2  VectorParamsAs1DForOutWhenUnconnected=off
  wires:
  Selector/1 -> "Rotation matrix in yaw "/1, Transposed rotation matrix in yaw1/1, Transposed rotation matrix in yaw/1
  Gain/1 -> Add2/1
  Demux1/1 -> Mux1/1
  Mux/1 -> eta_hat/1, Add1/2
  Gain1/1 -> Add4/1
  eta/1 -> Add/1, Selector/1
  Add3/1 -> Integrator2/1
  Gain7/1 -> Integrator3/1
  Integrator2/1 -> Gain6/1, Transposed rotation matrix in yaw1/2
  Gain8/1 -> Add6/3
  Integrator3/1 -> nu_hat/1, "Rotation matrix in yaw "/2, Gain8/1
  "Rotation matrix in yaw "/1 -> Add4/2
  Add5/1 -> Add6/2
  tau_est/1 -> Add5/2
  Gain6/1 -> Add3/2
  Mux1/1 -> Gain1/1, Gain2/1, Scope/1, Gain3/1, Gain/1
  Gain4/1 -> Add1/1
  Add2/1 -> Integrator1/1
  Demux1/2 -> Mux1/2
  "[-inf inf] to [-pi pi]"/1 -> Mux/3
  Gain2/1 -> Add3/1
  Gain5/1 -> Add2/2
  Add4/1 -> Integrator/1
  Demux/3 -> "[-inf inf] to [-pi pi]"/1
  Integrator1/1 -> Gain5/1, Gain4/1
  "[-inf inf] to [-pi pi]1"/1 -> Mux1/3
  Gain3/1 -> Transposed rotation matrix in yaw/2
  Transposed rotation matrix in yaw/1 -> Add5/1
  Add6/1 -> Gain7/1
  Integrator/1 -> Demux/1
  Add1/1 -> Add/2
  Add/1 -> Demux1/1
  Demux/2 -> Mux/2
  Demux1/3 -> "[-inf inf] to [-pi pi]1"/1
  Demux/1 -> Mux/1
  Transposed rotation matrix in yaw1/1 -> Add6/1

== system part2/Thrust Allocation/Subsystem ==
  alpha : Inport
  Demux : Demux  Outputs=5
  Mux : Mux  Inputs=5
  Unwrap : dspsigops/Unwrap  tol=pi  InputProcessing=Columns as channels (frame based)  running=off
  Unwrap1 : dspsigops/Unwrap  tol=pi  InputProcessing=Columns as channels (frame based)  running=off
  Unwrap2 : dspsigops/Unwrap  tol=pi  InputProcessing=Columns as channels (frame based)  running=off
  alpha [rad] : Outport
  wires:
  Demux/1 -> Mux/1
  Unwrap/1 -> Mux/5
  Mux/1 -> alpha [rad]/1
  Demux/5 -> Unwrap/1
  Unwrap1/1 -> Mux/4
  Demux/4 -> Unwrap1/1
  alpha/1 -> Demux/1
  Demux/2 -> Unwrap2/1
  Unwrap2/1 -> Mux/2
  Demux/3 -> Mux/3

== system part2/Wind/Subsystem ==
  angle : Inport
  C_pitch : Lookup_n-D  NumberOfTableDimensions=1  BreakpointsForDimension1=alpha  Table=C_pitch  InternalRulePriority=Speed  RndMeth=Simplest
  C_roll : Lookup_n-D  NumberOfTableDimensions=1  BreakpointsForDimension1=alpha  Table=C_roll  InternalRulePriority=Speed  RndMeth=Simplest
  C_yaw : Lookup_n-D  NumberOfTableDimensions=1  BreakpointsForDimension1=alpha  Table=C_yaw  InternalRulePriority=Speed  RndMeth=Simplest
  Cx : Lookup_n-D  NumberOfTableDimensions=1  BreakpointsForDimension1=alpha  Table=Cx  InternalRulePriority=Speed  RndMeth=Simplest
  Cy : Lookup_n-D  NumberOfTableDimensions=1  BreakpointsForDimension1=alpha  Table=Cy  InternalRulePriority=Speed  RndMeth=Simplest
  Cz : Lookup_n-D  NumberOfTableDimensions=1  BreakpointsForDimension1=alpha  Table=Cz  InternalRulePriority=Speed  RndMeth=Simplest
  Mux : Mux  Inputs=6
  Cw : Outport
  wires:
  Cx/1 -> Mux/1
  Mux/1 -> Cw/1
  angle/1 -> C_yaw/1, C_pitch/1, C_roll/1, Cz/1, Cy/1, Cx/1
  Cy/1 -> Mux/2
  Cz/1 -> Mux/3
  C_roll/1 -> Mux/4
  C_pitch/1 -> Mux/5
  C_yaw/1 -> Mux/6

== system part2/Wind/Wind speed ==
  Digital Clock : DigitalClock
  MATLAB Function : MATLAB Function  TreatAsAtomicUnit=on
  MATLAB Function1 : MATLAB Function  TreatAsAtomicUnit=on
  Scope : Scope
      settings: ActiveDisplayYMinimum=-4.98334  ActiveDisplayYMaximum=4.27891
  Scope1 : Scope
      settings: ActiveDisplayYMinimum=7.35139  ActiveDisplayYMaximum=9.35139  DataLoggingVariableName=ScopeData3
  Slow varying component : Subsystem
  Square : Math  Operator=square
  Sum : Sum  Inputs=+++
  U10 : Constant  Value=10
  Speed : Outport
  wires:
  U10/1 -> MATLAB Function1/2(U10), MATLAB Function/1(U10)
  Sum/1 -> Square/1
  Digital Clock/1 -> MATLAB Function1/1(t)  "Time"
  MATLAB Function1/1(U_gust) -> Sum/1, Scope/1
  MATLAB Function/1(U_mean) -> Scope1/1, Sum/2
  Slow varying component/1(Usv_dot) -> Sum/3
  Square/1 -> Speed/1

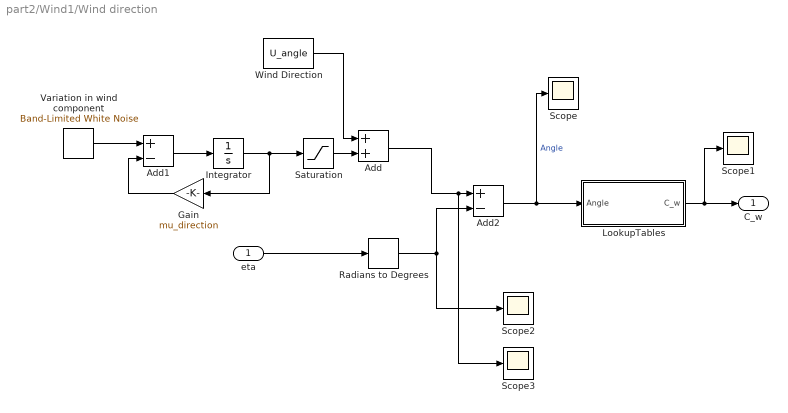
== system part2/Wind1/Wind direction ==
  eta : Inport
  Add : Sum
  Add1 : Sum  Inputs=+-
  Add2 : Sum  Inputs=+-
  Gain : Gain  Gain=mu_direction
  Integrator : Integrator
  LookupTables : Subsystem
  Radians to Degrees : simulink_extras/Transformations/Radians to Degrees
  Saturation : Saturate  UpperLimit=5  LowerLimit=-5
  Scope{,1..3} (4 alike) : Scope
      Scope settings: ActiveDisplayYMinimum=175.4013  ActiveDisplayYMaximum=184.40677
      Scope1 settings: ActiveDisplayYMinimum=-998.47601  ActiveDisplayYMaximum=2304.83067
      Scope2 settings: ActiveDisplayYMinimum=-0.05555  ActiveDisplayYMaximum=0.18675  DataLoggingVariableName=ScopeData4
      Scope3 settings: ActiveDisplayYMinimum=175.41243  ActiveDisplayYMaximum=184.57704  DataLoggingVariableName=ScopeData5
  Variation in wind component : simulink/Sources/Band-Limited White Noise  Cov=[0.15]  Ts=0.1  seed=[23381]
  Wind Direction : Constant  Value=U_angle
  C_w : Outport
  wires:
  eta/1 -> Radians to Degrees/1
  Wind Direction/1 -> Add/1
  Gain/1 -> Add1/2
  Add1/1 -> Integrator/1
  Variation in wind component/1 -> Add1/1
  Integrator/1 -> Saturation/1, Gain/1
  Add/1 -> Scope3/1, Add2/1
  Add2/1 -> LookupTables/1(Angle), Scope/1  "Angle"
  LookupTables/1(C_w) -> Scope1/1, C_w/1
  Saturation/1 -> Add/2
  Radians to Degrees/1 -> Scope2/1, Add2/2

== system part2/Wind1/Wind velocity components ==
  Add : Sum  Inputs=3
  Add1 : Sum  Inputs=+-
  Band-Limited White Noise : simulink/Sources/Band-Limited White Noise  Cov=[w]  Ts=0.1  seed=[23341]
  Constant : Constant  Value=U_mean
  Constant1 : Constant  Value=U_10
  Digital Clock : DigitalClock
  Gain : Gain  Gain=mu
  Integrator : Integrator
  MATLAB Function : MATLAB Function  TreatAsAtomicUnit=on
  Square : Math  Operator=square
  U_total : Outport
  wires:
  Add/1 -> Square/1
  Square/1 -> U_total/1
  Constant/1 -> Add/1  "U_mean"
  Add1/1 -> Integrator/1
  Band-Limited White Noise/1 -> Add1/1
  Integrator/1 -> Gain/1, Add/2  "USV"
  Gain/1 -> Add1/2
  Constant1/1 -> MATLAB Function/1(U_10)
  Digital Clock/1 -> MATLAB Function/2(t)
  MATLAB Function/1(U_gust) -> Add/3  "U_gust"

== system part2/Wind/Wind speed/Slow varying component ==
  Band-Limited White Noise : simulink/Sources/Band-Limited White Noise  Cov=[0.005]  Ts=0.1  seed=[23341]
  Integrator Limited : Integrator  LimitOutput=on  UpperSaturationLimit=1  LowerSaturationLimit=-1
  Sum1 : Sum  Inputs=|-+
  mu : Gain  Gain=0.001
  Usv_dot : Outport
  wires:
  Band-Limited White Noise/1 -> Sum1/2
  Sum1/1 -> Usv_dot/1, Integrator Limited/1  "Usv_dot"
  mu/1 -> Sum1/1
  Integrator Limited/1 -> mu/1  "Usv"

== system part2/Wind1/Wind direction/LookupTables ==
  Angle : Inport
  1-D Lookup Table : Lookup_n-D  NumberOfTableDimensions=1  BreakpointsForDimension1=wind_coeff(:,1)  Table=wind_coeff(:,2)  InternalRulePriority=Speed  RndMeth=Simplest
  1-D Lookup Table1 : Lookup_n-D  NumberOfTableDimensions=1  BreakpointsForDimension1=wind_coeff(:,1)  Table=wind_coeff(:,3)  InternalRulePriority=Speed  RndMeth=Simplest
  1-D Lookup Table2 : Lookup_n-D  NumberOfTableDimensions=1  BreakpointsForDimension1=wind_coeff(:,1)  Table=wind_coeff(:,4)  InternalRulePriority=Speed  RndMeth=Simplest
  1-D Lookup Table3 : Lookup_n-D  NumberOfTableDimensions=1  BreakpointsForDimension1=wind_coeff(:,1)  Table=wind_coeff(:,5)  InternalRulePriority=Speed  RndMeth=Simplest
  1-D Lookup Table4 : Lookup_n-D  NumberOfTableDimensions=1  BreakpointsForDimension1=wind_coeff(:,1)  Table=wind_coeff(:,6)  InternalRulePriority=Speed  RndMeth=Simplest
  1-D Lookup Table5 : Lookup_n-D  NumberOfTableDimensions=1  BreakpointsForDimension1=wind_coeff(:,1)  Table=wind_coeff(:,7)  InternalRulePriority=Speed  RndMeth=Simplest
  Mux : Mux  Inputs=6
  C_w : Outport
  wires:
  Angle/1 -> 1-D Lookup Table2/1, 1-D Lookup Table1/1, 1-D Lookup Table/1, 1-D Lookup Table3/1, 1-D Lookup Table4/1, 1-D Lookup Table5/1
  Mux/1 -> C_w/1
  1-D Lookup Table/1 -> Mux/1
  1-D Lookup Table1/1 -> Mux/2
  1-D Lookup Table2/1 -> Mux/3
  1-D Lookup Table3/1 -> Mux/4
  1-D Lookup Table4/1 -> Mux/5
  1-D Lookup Table5/1 -> Mux/6

== matlab function part2/Observer/Extended kalmanfilter/Kalman Corrector ==
  data: x_hat output; P_hat output; eta input; x_pred input; P_pred input; H_ekf parameter; R_ekf parameter
function [x_hat, P_hat] = fcn(eta, x_pred, P_pred, H_ekf, R_ekf)
%where x_est and P_est is the state observer

Kalman_gain = P_pred*H_ekf'*inv(H_ekf*P_pred*H_ekf'+R_ekf);
P_hat = (eye(15)-Kalman_gain*H_ekf)*P_pred*(eye(15)-Kalman_gain*H_ekf)'+Kalman_gain*R_ekf*Kalman_gain';
x_hat = x_pred+Kalman_gain*(eta-H_ekf*x_pred);

end

== matlab function part2/Wind1/Wind velocity components/MATLAB Function ==
  data: U_10 input; U_gust output; t input
function U_gust = fcn(U_10, t)
    % Parameters based on lecture notes
    L = 1800; % [m]
    K = 0.0026;
    f = linspace(0.0001, 1, 500);
    N = length(f);
    delta_f = f(2) - f(1);
    U_gust = zeros(size(t));
    
    for i= 1:N
        f_tilde = (L*f(i))/U_10;
        S = (4*K*L*U_10)./((2+f_tilde.^2).^(5/6));
        phi = rand(1) * 2 * pi; % Random phase
        U_gust = U_gust + sqrt(2*S*delta_f)*cos(2*pi*f(i)*t+phi);
    end
end

== matlab function part2/Thrust Allocation/MATLAB Function1 ==
  data: tau input; u output; B input; alpha output
function [u, alpha] = fcn(tau, B)
    % Dimensions
    % u - [1x5]
    % alpha - [1x5]
    % tau - [surge, sway, yaw] from PID
    % B - [3x8]
    
    % Initial thrust
    Td0 = zeros(8,1);

    % Previously measured u 
    persistent u_l
    
    if isempty(u_l)
        u_l = Td0;
    end

    %% Define rudder saturation and rotation limitation
    u_max = 10.*[125000, ones(1,2)*150000, 125000, ones(1,2)*300000, ones(1,2)*300000]';
    u_min = -u_max;
    
    % Rate of thruster power
    h = 0.1;
    delta_max = 10.*[125000/8*h, ones(1,2)*150000/8*h, 125000/8*h, ones(1,2)*300000/10*h,ones(1,2)*300000/10*h]';
    delta_min = -delta_max;
    
    % Constraint
    lim_max = delta_max + u_l;
    lim_min = delta_min + u_l;
    
    % Weight matrix 2*diag(m,m,m,m,m ..., p..)
    % (t1, a1y, a1x, t2, a2y, a2x, a3y, a3x,...)
    H =  2*diag([1,0.8,0.8,1,0.8,0.8,0.8,0.8,1e4,1e4,1e5]); 

    % A og Aequality
    A_eq = [B, -eye(3)];
    A = [-eye(8) ,  zeros(8,3);
      eye(8) ,   zeros(8,3)];
    
    % b og bequality
    b_eq = [tau(1), tau(2), tau(6)];
    b = [-(max(u_min, lim_min)); 
           min(u_max,lim_max)];
    
    coder.extrinsic('quadprog');
    coder.extrinsic('optimoptions');
    options = optimoptions('quadprog',...
     'Algorithm','interior-point-convex','Display','off','Steptolerance',...
    1e-30,'OptimalityTolerance',1e+3);

    x = ones(11,1);
    f = zeros(length(H),1);

    x = quadprog(H,f,A,b,A_eq,b_eq, [],[],[],options);
    Td = x(1:8);
   
    uy_aft = Td(5)+Td(7);

    u04 = -10;
    u05 = 10;

    % ensuring no inline flow on aft propellers
    if uy_aft >= 0
        u4y = u04;
        u5y = uy_aft+u05;
    else 
        u4y = uy_aft+u04;
        u5y = u05;
    end

    u1 = Td(1);
    u2 = sqrt(Td(2)^2+Td(3)^2);
    u3 = Td(4);

    u4x = Td(6);
    u5x = Td(8);

    u4 = sqrt(u4x^2+u4y^2);
    u5 = sqrt(u5x^2+u5y^2);
    
    a1 = pi/2;
    a2 = atan2(Td(2),Td(3));
    a3 = pi/2;
    a4 = atan2(u4y,u4x);
    a5 = atan2(u5y,u5x);
    
    u_l = Td(1:8);
    
    alpha = [a1 a2 a3 a4 a5]';
    u = [u1 u2 u3 u4 u5]';

== matlab function part2/Thrust Allocation/MATLAB Function ==
  data: tau_d input; u1 output; xpos input; ypos input; alpha output; thrust input; rate input; rotationspeed input; W input; xprev input; aprev input; uprev input; xnew output
function [u1,alpha,xnew] = fcn(tau_d, xpos, ypos, thrust, rate, rotationspeed, W, xprev, aprev, uprev)
l_1 = xpos(1);
l_2x = xpos(2);
l_2y = ypos(2);
l_3 = xpos(3);
l_4x = xpos(4);
l_4y = ypos(4);
l_5x = xpos(5);
l_5y = ypos(5);
B = [[0, 1, 0, 0, 1, 0, 1, 0];
    [1, 0, 1, 1, 0, 1, 0, 1];
    [l_1, l_2y, l_2x, l_3, l_4y, l_4x, l_5y, l_5x]];


if ~isequal(size(tau_d), [3, 1])
    beq=[0 0 0];
else
    beq=tau_d;
end

thrusterfault = 0;
if thrusterfault==1
    B=[[0, 0, 0, 0, 0, 0, 1, 0];
    [1, 0, 0, 1, 0, 0, 0, 1];
    [l_1, 0, 0, l_3, 0, 0, l_5y, l_5x]];
end
s = zeros(3,1);
%Variables used in quadprog'
H = blkdiag(W, 10000*eye(length(s)));
f = zeros(11, 1);
%Constraints for quadprog
Aeq = [B, -eye(3)];
max_thrust=min(thrust, xprev+rate);
min_thrust=max(-thrust, xprev-rate);
A = [-eye(8), zeros(8, 3);
    eye(8), zeros(8, 3);];
    % 0 0 0 0 -tan(maxangle4) 1 0 0 0 0 0;
    % 0 0 0 0 tan(minangle4) -1 0 0 0 0 0;
    % 0 0 0 0 0 0 -tan(maxangle5) 1 0 0 0;
    % 0 0 0 0 0 0 tan(minangle5) -1 0 0 0];
b = [-min_thrust; max_thrust];% zeros(4,1)];
x0 = zeros(11, 1);
options = optimoptions('quadprog', 'Algorithm', 'active-set', 'Display', 'off');
x = quadprog(H,f, A, b, Aeq, beq,[], [], x0, options);
alpha1=zeros(5,1);
alpha1(1) = pi/2;
alpha1(2) = atan2(x(3), x(2));
alpha1(3)= pi/2;
alpha1(4)= atan2(x(6), x(5));
alpha1(5)= atan2(x(8), x(7));
u=zeros(1,5);
u(1)=x(1);
u(2)=sqrt(x(2)^2 + x(3)^2);
u(3)=x(4);
u(4)=sqrt(x(5)^2 + x(6)^2);
u(5)=sqrt(x(7)^2 + x(8)^2);
xnew=x(1:8);
%change limitation
change2 = wrapToPi(alpha1(2) - aprev(2));
change4 = wrapToPi(alpha1(4) - aprev(4));
change5 = wrapToPi(alpha1(5) - aprev(5));
changeArr=zeros(1,5);
changeArr(2)=change2;
changeArr(4)=change4;
changeArr(5)=change5;
%Forbidden zones
%%Constraint in total
for i = [2, 4, 5]
    if u(i) > thrust(i)
        u(i) = thrust(i);
    end
    if abs(changeArr(i)) > rotationspeed(i)
        if changeArr(i) < 0
            changeArr(i) = -rotationspeed(i);
        else
            changeArr(i) = rotationspeed(i);
        end
        alpha1(i)=aprev(i)+changeArr(i);
    end
end
%Forbidden zones thruster 2
% if pi/8 <= alpha1(2) && alpha1(2) > -pi/8
%     alpha1(2) = pi/8;
% end
%Forbidden zones thruster 4
if -7*pi/8 >= alpha1(4) || alpha1(4) > 7*pi/8
    alpha1(4) = -7*pi/8;
end
if -7*pi/8 >= alpha1(4)&& alpha1(4)>= -pi
    alpha1(4) = -7*pi/8;
end
if pi >= alpha1(4) && alpha1(4)>= 7*pi/8
    alpha1(4) = 7*pi/8;
end
%Forbidden zones thruster 5
if -7*pi/8 >= alpha1(5)&& alpha1(5)>= -pi
    alpha1(5) = -7*pi/8;
end
if pi >= alpha1(5) && alpha1(5)>= 7*pi/8
    alpha1(5) = 7*pi/8;
end

if thrusterfault == 0
    if 3*pi/8 <= alpha1(4) && alpha1(4) <=4*pi/8
       alpha1(4) = 3*pi/8;
    end
    if 4*pi/8 <= alpha1(4) && alpha1(4) <=5*pi/8
       alpha1(4) = 5*pi/8;
    end
    if -4*pi/8 >= alpha1(5) && alpha1(5) < -5*pi/8
       alpha1(5) = -5*pi/8;
    end
    if -3*pi/8 >= alpha1(5) && alpha1(5) <= -4*pi/8
       alpha1(5) = -3*pi/8;
    end
end
%Lets start again
Bnew=[0   cos(alpha1(2))      0   cos(alpha1(4))                            cos(alpha1(5));
      1   sin(alpha1(2))      1   sin(alpha1(4))                            sin(alpha1(5));
      l_1 l_2x*sin(alpha1(2)) l_3 l_4x*sin(alpha1(4)) + l_4y*cos(alpha1(4)) l_5x*sin(alpha1(5)) + l_5y*cos(alpha1(5))];
if thrusterfault==1
    Bnew=[0   0      0   0 cos(alpha1(5));
      1   0      1   0 sin(alpha1(5));
      l_1 0 l_3 0 l_5x*sin(alpha1(5)) + l_5y*cos(alpha1(5))];
end
%Variables used in quadprog'
newW=diag([10,8,10,8,8]);
newH = blkdiag(newW, 10000*eye(length(s)));
newf = zeros(8, 1);
%Constraints for new quadprog
newAeq = [Bnew, -eye(3)];
newthrust=zeros(5, 1);
newthrust(1)=thrust(1);
newthrust(2)=thrust(2);
newthrust(3)=thrust(4);
newthrust(4)=thrust(5);
newthrust(5)=thrust(7);
newrate=zeros(5, 1);
newrate(1)=rate(1);
newrate(2)=rate(2);
newrate(3)=rate(4);
newrate(4)=rate(5);
newrate(5)=rate(7);
newmax_thrust=min(newthrust, uprev+newrate);
newmin_thrust=max(-newthrust, uprev-newrate);
newA = [-eye(5), zeros(5, 3);
    eye(5), zeros(5, 3)];
newb = [-newmin_thrust; newmax_thrust];
newx0 = zeros(8, 1);
newoptions = optimoptions('quadprog', 'Algorithm', 'active-set', 'Display', 'off');
x2 = quadprog(newH,newf, newA, newb, newAeq, beq,[], [], newx0, newoptions);
u1=x2(1:5);
alpha=alpha1;
end

== matlab function part2/Wind/Wind speed/MATLAB Function1 ==
  settings: updateMethod=DISCRETE
  data: t input; U10 input; U_gust output
function U_gust = fcn(t, U10)
    % Parameters based on lecture notes
    L = 1800; % [m]
    K = 0.0026;
    f = linspace(0.0001, 1, 500);
    N = length(f);
    delta_f = f(2) - f(1);
    U_gust = zeros(size(t));
    for i= 1:N
        f_tilde = (L*f(i))/U10;
        S = (4 * K * L * U10)./((2+f_tilde.^2).^(5/6));
        phi = rand(1) * 2 * pi; 
        U_gust = U_gust + sqrt(2*S*delta_f)*cos(2*pi*f(i)*t+phi);
    end
end

== matlab function part2/Wind/Wind speed/MATLAB Function ==
  data: U10 input; U_mean output
function U_mean = fcn(U10)

K = 0.003;
z = 3;
z0 = 10*exp(-2/(5*sqrt(K)));

U_mean = U10*(5/2)*sqrt(K)*log(z/z0);

end

== matlab function part2/Thruster Dynamics/MATLAB Function ==
  data: alpha_actual input; thrust_actual input; actual_tau output; PosX input; PosY input
function actual_tau   = fcn(alpha_actual,thrust_actual,PosX,PosY)

    Alpha_surge =[cos(alpha_actual(1)) cos(alpha_actual(2)) cos(alpha_actual(3)) cos(alpha_actual(4)) cos(alpha_actual(5))];  
    Alpha_sway = [sin(alpha_actual(1)) sin(alpha_actual(2)) sin(alpha_actual(3)) sin(alpha_actual(4)) sin(alpha_actual(5))];
    Alpha_yaw = [sin(alpha_actual(1))*PosX(1)-cos(alpha_actual(1))*PosY(1) sin(alpha_actual(2))*PosX(2)-cos(alpha_actual(2))*PosY(2) ...
                 sin(alpha_actual(3))*PosX(3)-cos(alpha_actual(3))*PosY(3) sin(alpha_actual(4))*PosX(4)-cos(alpha_actual(4))*PosY(4) ...
                 sin(alpha_actual(5))*PosX(5)-cos(alpha_actual(5))*PosY(5)];

    actual_tau = [Alpha_surge; Alpha_sway; Alpha_yaw]*thrust_actual;
end
